simulink model "roll_ap_rev"  (R2021b)
settings: Solver=FixedStepDiscrete  StartTime=0.0  StopTime=25  FixedStep=1/40  RelTol=1e-3
model workspace (MAT data in the model file):
  AP_Eng = [1 1 1 1 1 1 1 1 1 1 1 1 ... (1001 elements, 1001x1)]
  Ail_cmd = [0 -0.149968761714 -0.301000114013 -0.452906745732 -0.6055025668 -0.758604051758 -0.912031519861 -1.0656103303 -1.21917197401 -1.37255504699 -1.52560609378 -1.67818031361 ... (1001 elements, 1001x1)]
  FR = [0; 0; 0; 0; 0; 0]
  HDG_Mode = [0 0 0 0 0 0 0 0 0 0 0 0 ... (1001 elements, 1001x1)]
  HDG_Ref = [0 0 0 0 0 0 0 0 0 0 0 0 ... (1001 elements, 1001x1)]
  InputSize = 6
  N = 28
  P = [0 0 0 0 0 0 0 0 0 0 0 0 ... (1001 elements, 1001x1)]
  Phi = [0 0.0499895872378 0.0999167914439 0.149719695422 0.199337304982 0.248709989094 0.297779895219 0.346491332905 0.3947911197 0.442628884696 0.489957326254 0.536732421812 ... (1001 elements, 1001x1)]
  Psi = [0 0 0 0 0 0 0 0 0 0 0 0 ... (1001 elements, 1001x1)]
  TAS = [0 0 0 0 0 0 0 0 0 0 0 0 ... (1001 elements, 1001x1)]
  TimeSteps = 1001
  TurnK = [0 0 0 0 0 0 0 0 0 0 0 0 ... (1001 elements, 1001x1)]
  X = [-123.259290596  -128.902651481  56.0666516964  743.094931803  83.0616505427  1  -22.0520305237  -100.36159472; 167.816750695  -28.1659382545  59.9981123607  743.132468125  0  1  -48.3367940279  -4.89724193602; 164.580101367  -126.393552121  54.8898007227  346.111605096  0  11.0421280531  95.5860437336  13.049515342; -5.26476645978  105.176372028  156.237569193  657.090475075  0  1  106.271964409  18.5100430761; 109.697619539  165.417273501  -162.797252325  171.186687812  0  1  -112.72586236  193.817894952; -123.259290596  147.137423095  126.863401086  757.740130578  0  1  -22.0520305237  -15.0695729805]
  curPath = '/Users/khouloud.gaaloul/Documents/Projects/QRA-Search/Problems/SimulinkTesting'
  dispGain = Simulink.Parameter
  dispGain.Value = 1
  dispGain.DataType = 'auto'
  dispGain.Complexity = 'real'
  dispGain.Dimensions = [1 1]
  hdgGain = Simulink.Parameter
  hdgGain.Value = 0.015
  hdgGain.DataType = 'auto'
  hdgGain.Min = 0
  hdgGain.Complexity = 'real'
  hdgGain.Dimensions = [1 1]
  hws : handle (value not decoded)
  i = 17
  intGain = Simulink.Parameter
  intGain.Value = 1
  intGain.DataType = 'auto'
  intGain.Complexity = 'real'
  intGain.Dimensions = [1 1]
  j = 4
  list(1).name = 'AP_Eng'
  list(1).size = [1001 1]
  list(1).bytes = 1001
  list(1).class = 'logical'
  list(1).global = 0
  list(1).sparse = 0
  list(1).complex = 0
  list(1).nesting.function = 'simroll_ap'
  list(1).nesting.level = 1
  list(1).persistent = 0
  list(2).name = 'Ail_cmd'
  list(2).size = [1001 1]
  list(2).bytes = 8008
  list(2).class = 'double'
  list(2).global = 0
  list(2).sparse = 0
  list(2).complex = 0
  list(2).nesting.function = 'simroll_ap'
  list(2).nesting.level = 1
  list(2).persistent = 0
  list(3).name = 'FR'
  list(3).size = [6 1]
  list(3).bytes = 48
  list(3).class = 'double'
  list(3).global = 0
  list(3).sparse = 0
  list(3).complex = 0
  list(3).nesting.function = 'simroll_ap'
  list(3).nesting.level = 1
  list(3).persistent = 0
  list(4).name = 'HDG_Mode'
  list(4).size = [1001 1]
  list(4).bytes = 1001
  list(4).class = 'logical'
  list(4).global = 0
  list(4).sparse = 0
  list(4).complex = 0
  list(4).nesting.function = 'simroll_ap'
  list(4).nesting.level = 1
  list(4).persistent = 0
  list(5).name = 'HDG_Ref'
  list(5).size = [1001 1]
  list(5).bytes = 8008
  list(5).class = 'double'
  list(5).global = 0
  list(5).sparse = 0
  list(5).complex = 0
  list(5).nesting.function = 'simroll_ap'
  list(5).nesting.level = 1
  list(5).persistent = 0
  list(6).name = 'InputSize'
  list(6).size = [1 1]
  list(6).bytes = 8
  list(6).class = 'double'
  list(6).global = 0
  list(6).sparse = 0
  list(6).complex = 0
  list(6).nesting.function = 'simroll_ap'
  list(6).nesting.level = 1
  list(6).persistent = 0
  list(7).name = 'N'
  list(7).size = [1 1]
  list(7).bytes = 8
  list(7).class = 'double'
  list(7).global = 0
  list(7).sparse = 0
  list(7).complex = 0
  list(7).nesting.function = 'simroll_ap'
  list(7).nesting.level = 1
  list(7).persistent = 0
  list(8).name = 'P'
  list(8).size = [1001 1]
  list(8).bytes = 8008
  list(8).class = 'double'
  list(8).global = 0
  list(8).sparse = 0
  list(8).complex = 0
  list(8).nesting.function = 'simroll_ap'
  list(8).nesting.level = 1
  list(8).persistent = 0
  list(9).name = 'Phi'
  list(9).size = [1001 1]
  list(9).bytes = 8008
  list(9).class = 'double'
  list(9).global = 0
  list(9).sparse = 0
  list(9).complex = 0
  list(9).nesting.function = 'simroll_ap'
  list(9).nesting.level = 1
  list(9).persistent = 0
  list(10).name = 'Psi'
  list(10).size = [1001 1]
  list(10).bytes = 8008
  list(10).class = 'double'
  list(10).global = 0
  list(10).sparse = 0
  list(10).complex = 0
  list(10).nesting.function = 'simroll_ap'
  list(10).nesting.level = 1
  list(10).persistent = 0
  list(11).name = 'TAS'
  list(11).size = [1001 1]
  list(11).bytes = 8008
  list(11).class = 'double'
  list(11).global = 0
  list(11).sparse = 0
  list(11).complex = 0
  list(11).nesting.function = 'simroll_ap'
  list(11).nesting.level = 1
  list(11).persistent = 0
  list(12).name = 'TimeSteps'
  list(12).size = [1 1]
  list(12).bytes = 8
  list(12).class = 'double'
  list(12).global = 0
  list(12).sparse = 0
  list(12).complex = 0
  list(12).nesting.function = 'simroll_ap'
  list(12).nesting.level = 1
  list(12).persistent = 0
  list(13).name = 'TurnK'
  list(13).size = [1001 1]
  list(13).bytes = 8008
  list(13).class = 'double'
  list(13).global = 0
  list(13).sparse = 0
  list(13).complex = 0
  list(13).nesting.function = 'simroll_ap'
  list(13).nesting.level = 1
  list(13).persistent = 0
  list(14).name = 'X'
  list(14).size = [6 8]
  list(14).bytes = 384
  list(14).class = 'double'
  list(14).global = 0
  list(14).sparse = 0
  list(14).complex = 0
  list(14).nesting.function = 'simroll_ap'
  list(14).nesting.level = 1
  list(14).persistent = 0
  list(15).name = 'curPath'
  list(15).size = [1 78]
  list(15).bytes = 156
  list(15).class = 'char'
  list(15).global = 0
  list(15).sparse = 0
  list(15).complex = 0
  list(15).nesting.function = 'simroll_ap'
  list(15).nesting.level = 1
  list(15).persistent = 0
  list(16).name = 'hws'
  list(16).size = [1 1]
  list(16).bytes = 0
  list(16).class = 'Simulink.ModelWorkspace'
  list(16).global = 0
  list(16).sparse = 0
  list(16).complex = 0
  list(16).nesting.function = 'simroll_ap'
  list(16).nesting.level = 1
  list(16).persistent = 0
  list(17).name = 'i'
  list(17).size = [1 1]
  list(17).bytes = 8
  list(17).class = 'double'
  list(17).global = 0
  list(17).sparse = 0
  list(17).complex = 0
  list(17).nesting.function = 'simroll_ap'
  list(17).nesting.level = 1
  list(17).persistent = 0
  list(18).name = 'j'
  list(18).size = [1 1]
  list(18).bytes = 8
  list(18).class = 'double'
  list(18).global = 0
  list(18).sparse = 0
  list(18).complex = 0
  list(18).nesting.function = 'simroll_ap'
  list(18).nesting.level = 1
  list(18).persistent = 0
  list(19).name = 'list'
  list(19).size = [28 1]
  list(19).bytes = 40880
  list(19).class = 'struct'
  list(19).global = 0
  list(19).sparse = 0
  list(19).complex = 0
  list(19).nesting.function = 'simroll_ap'
  list(19).nesting.level = 1
  list(19).persistent = 0
  list(20).name = 'modelpath'
  list(20).size = [1 95]
  list(20).bytes = 190
  list(20).class = 'char'
  list(20).global = 0
  list(20).sparse = 0
  list(20).complex = 0
  list(20).nesting.function = 'simroll_ap'
  list(20).nesting.level = 1
  list(20).persistent = 0
  list(21).name = 'models'
  list(21).size = [1 4]
  list(21).bytes = 1328
  list(21).class = 'cell'
  list(21).global = 0
  list(21).sparse = 0
  list(21).complex = 0
  list(21).nesting.function = 'simroll_ap'
  list(21).nesting.level = 1
  list(21).persistent = 0
  list(22).name = 'n'
  list(22).size = [1 1]
  list(22).bytes = 8
  list(22).class = 'double'
  list(22).global = 0
  list(22).sparse = 0
  list(22).complex = 0
  list(22).nesting.function = 'simroll_ap'
  list(22).nesting.level = 1
  list(22).persistent = 0
  list(23).name = 'nbrInputs'
  list(23).size = [1 1]
  list(23).bytes = 8
  list(23).class = 'double'
  list(23).global = 0
  list(23).sparse = 0
  list(23).complex = 0
  list(23).nesting.function = 'simroll_ap'
  list(23).nesting.level = 1
  list(23).persistent = 0
  list(24).name = 'rollIn'
  list(24).size = [1 1]
  list(24).bytes = 60394
  list(24).class = 'struct'
  list(24).global = 0
  list(24).sparse = 0
  list(24).complex = 0
  list(24).nesting.function = 'simroll_ap'
  list(24).nesting.level = 1
  list(24).persistent = 0
  list(25).name = 'rollOut'
  list(25).size = [1 1]
  list(25).bytes = 17110
  list(25).class = 'struct'
  list(25).global = 0
  list(25).sparse = 0
  list(25).complex = 0
  list(25).nesting.function = 'simroll_ap'
  list(25).nesting.level = 1
  list(25).persistent = 0
  list(26).name = 's1'
  list(26).size = [1 1001]
  list(26).bytes = 8008
  list(26).class = 'double'
  list(26).global = 0
  list(26).sparse = 0
  list(26).complex = 0
  list(26).nesting.function = 'simroll_ap'
  list(26).nesting.level = 1
  list(26).persistent = 0
  list(27).name = 'simOut'
  list(27).size = [1 1]
  list(27).bytes = 23416
  list(27).class = 'Simulink.SimulationOutput'
  list(27).global = 0
  list(27).sparse = 0
  list(27).complex = 0
  list(27).nesting.function = 'simroll_ap'
  list(27).nesting.level = 1
  list(27).persistent = 0
  list(28).name = 't'
  list(28).size = [1 1001]
  list(28).bytes = 8008
  list(28).class = 'double'
  list(28).global = 0
  list(28).sparse = 0
  list(28).complex = 0
  list(28).nesting.function = 'simroll_ap'
  list(28).nesting.level = 1
  list(28).persistent = 0
  modelpath = '/Users/khouloud.gaaloul/Documents/Projects/QRA-Search/SimulinkModels/autopilot_R2013b_workarea/'
  models = {'/Users/khouloud.gaaloul/Documents/Projects/QRA-Search/SimulinkModels/autopilot_R2013b_workarea/AP_Lib.slx', '/Users/khouloud.gaaloul/Documents/Projects/QRA-Search/SimulinkModels/autopilot_R2013b_workarea/Heading_Mode.slx', '/Users/khouloud.gaaloul/Documents/Projects/QRA-Search/SimulinkModels/autopilot_R2013b_workarea/attitude_controller.slx', '/Users/khouloud.gaaloul/Documents/Projects/QRA-Search/SimulinkModels/autopilot_R2013b_workarea/roll_ap.slx'}
  n = 6
  nbrInputs = 8
  rateGain = Simulink.Parameter
  rateGain.Value = 3
  rateGain.DataType = 'auto'
  rateGain.Complexity = 'real'
  rateGain.Dimensions = [1 1]
  rollIn.signals(1).values = [0 0.0499895872378 0.0999167914439 0.149719695422 0.199337304982 0.248709989094 0.297779895219 0.346491332905 0.3947911197 0.442628884696 0.489957326254 0.536732421812 ... (1001 elements, 1001x1)]
  rollIn.signals(1).dimensions = 1
  rollIn.signals(2).values = [0 0 0 0 0 0 0 0 0 0 0 0 ... (1001 elements, 1001x1)]
  rollIn.signals(2).dimensions = 1
  rollIn.signals(3).values = [0 0 0 0 0 0 0 0 0 0 0 0 ... (1001 elements, 1001x1)]
  rollIn.signals(3).dimensions = 1
  rollIn.signals(4).values = [0 0 0 0 0 0 0 0 0 0 0 0 ... (1001 elements, 1001x1)]
  rollIn.signals(4).dimensions = 1
  rollIn.signals(5).values = [1 1 1 1 1 1 1 1 1 1 1 1 ... (1001 elements, 1001x1)]
  rollIn.signals(5).dimensions = 1
  rollIn.signals(6).values = [0 0 0 0 0 0 0 0 0 0 0 0 ... (1001 elements, 1001x1)]
  rollIn.signals(6).dimensions = 1
  rollIn.signals(7).values = [0 0 0 0 0 0 0 0 0 0 0 0 ... (1001 elements, 1001x1)]
  rollIn.signals(7).dimensions = 1
  rollIn.signals(8).values = [0 0 0 0 0 0 0 0 0 0 0 0 ... (1001 elements, 1001x1)]
  rollIn.signals(8).dimensions = 1
  rollIn.time = [0 0.025 0.05 0.075 0.1 0.125 0.15 0.175 0.2 0.225 0.25 0.275 ... (1001 elements, 1001x1)]
  rollOut.time = [0 0.025 0.05 0.075 0.1 0.125 0.15 0.175 0.2 0.225 0.25 0.275 ... (1001 elements, 1001x1)]
  rollOut.signals.values = [0 -0.149968761714 -0.301000114013 -0.452906745732 -0.6055025668 -0.758604051758 -0.912031519861 -1.0656103303 -1.21917197401 -1.37255504699 -1.52560609378 -1.67818031361 ... (1001 elements, 1001x1)]
  rollOut.signals.dimensions = 1
  rollOut.signals.label = ''
  rollOut.signals.blockName = 'roll_ap/Ail Cmd'
  s1 = [-123.259290596 -123.259290596 -123.259290596 -123.259290596 -123.259290596 -123.259290596 -123.259290596 -123.259290596 -123.259290596 -123.259290596 -123.259290596 -123.259290596 ... (1001 elements, 1x1001)]
  s5 = [0 0 0 0 0 0 0 0 0 0 0 0 ... (1001 elements, 1x1001)]
  simOut = Simulink.SimulationOutput
  simOut.Data.rollOut.time = [0 0.025 0.05 0.075 0.1 0.125 0.15 0.175 0.2 0.225 0.25 0.275 ... (1001 elements, 1001x1)]
  simOut.Data.rollOut.signals.values = [0 -0.149968761714 -0.301000114013 -0.452906745732 -0.6055025668 -0.758604051758 -0.912031519861 -1.0656103303 -1.21917197401 -1.37255504699 -1.52560609378 -1.67818031361 ... (1001 elements, 1001x1)]
  simOut.Data.rollOut.signals.dimensions = 1
  simOut.Data.rollOut.signals.label = ''
  simOut.Data.rollOut.signals.blockName = 'roll_ap/Ail Cmd'
  simOut.Metadata = Simulink.SimulationMetadata
  simOut.Metadata.ModelInfo.ModelName = 'roll_ap'
  simOut.Metadata.ModelInfo.ModelVersion = '1.169'
  simOut.Metadata.ModelInfo.ModelFilePath = '/Users/khouloud.gaaloul/Documents/Projects/QRA-Search/SimulinkModels/autopilot_R2013b_workarea/roll_ap.slx'
  simOut.Metadata.ModelInfo.UserID = 'khouloud.gaaloul'
  simOut.Metadata.ModelInfo.MachineName = ''
  simOut.Metadata.ModelInfo.Platform = 'MACI64'
  simOut.Metadata.ModelInfo.ModelStructuralChecksum = [2583199931; 2424133270; 1270005224; 292482032]
  simOut.Metadata.ModelInfo.SimulationMode = 'normal'
  simOut.Metadata.ModelInfo.StartTime = 0
  simOut.Metadata.ModelInfo.StopTime = 25
  simOut.Metadata.ModelInfo.SolverInfo.Type = 'Fixed-Step'
  simOut.Metadata.ModelInfo.SolverInfo.Solver = 'FixedStepDiscrete'
  simOut.Metadata.ModelInfo.SolverInfo.FixedStepSize = 0.025
  simOut.Metadata.ModelInfo.SimulinkVersion.Name = 'Simulink'
  simOut.Metadata.ModelInfo.SimulinkVersion.Version = '8.7'
  simOut.Metadata.ModelInfo.SimulinkVersion.Release = '(R2016a)'
  simOut.Metadata.ModelInfo.SimulinkVersion.Date = '10-Feb-2016'
  simOut.Metadata.TimingInfo.WallClockTimestampStart = '2018-03-29 14:31:33.008650'
  simOut.Metadata.TimingInfo.WallClockTimestampStop = '2018-03-29 14:31:35.732856'
  simOut.Metadata.TimingInfo.InitializationElapsedWallTime = 2.646185
  simOut.Metadata.TimingInfo.ExecutionElapsedWallTime = 0.010666
  simOut.Metadata.TimingInfo.TerminationElapsedWallTime = 0.067366
  simOut.Metadata.TimingInfo.TotalElapsedWallTime = 2.724217
  simOut.Metadata.ExecutionInfo.StopEvent = 'ReachedStopTime'
  simOut.Metadata.ExecutionInfo.StopEventSource = []
  simOut.Metadata.ExecutionInfo.StopEventDescription = 'Reached stop time of 25'
  simOut.Metadata.ExecutionInfo.ErrorDiagnostic = []
  simOut.Metadata.ExecutionInfo.WarningDiagnostics = struct([])
  simOut.Metadata.AppInfo = struct()
  t = [0 0.025 0.05 0.075 0.1 0.125 0.15 0.175 0.2 0.225 0.25 0.275 ... (1001 elements, 1x1001)]
libraries: simulink x2
(part 1 of 2)
settings Model: RequirementInfo={} %GIDa_fe9045fd_0412_4b6e_8206_617cc20e6fde  ParameterArgumentNames=dispGain,intGain,rateGain,hdgGain  Creator=bpotter  LastModifiedBy=achan260
settings SolverCC: AlgebraicLoopSolver=TrustRegion
settings DataIOCC: ExternalInput=rollIn  LoadExternalInput=on  SaveFormat=StructureWithTime  SaveOutput=off  DSMLogging=off  SaveTime=off  ReturnWorkspaceOutputs=off  OutputSaveName=Ail_Cmd  SignalLoggingName=roll_ap_logsout
settings OptimizationCC: BlockReduction=off  DefaultParameterBehavior=Inlined  InlineInvariantSignals=on  ExpressionDepthLimit=2147483647  EfficientFloat2IntCast=on  EfficientMapNaN2IntZero=off  LifeSpan=inf  MaxStackSize=inf  EfficientTunableParamExpr=on
settings DebuggingCC: SignalInfNanChecking=error  SignalRangeChecking=error  ReadBeforeWriteMsg=EnableAllAsError  WriteAfterWriteMsg=EnableAllAsError  WriteAfterReadMsg=EnableAllAsError  AlgebraicLoopMsg=error  ArtificialAlgebraicLoopMsg=error  SaveWithDisabledLinksMsg=error  SaveWithParameterizedLinksMsg=error  CheckExecutionContextPreStartOutputMsg=on  BlockPriorityViolationMsg=error  MaxConsecutiveZCsMsg=warning  SolverPrmCheckMsg=error  InheritedTsInSrcMsg=error  SingleTaskRateTransMsg=error  TasksWithSamePriorityMsg=error  SigSpecEnsureSampleTimeMsg=error  CheckMatrixSingularityMsg=error  IntegerOverflowMsg=error  ParameterUnderflowMsg=error  ParameterPrecisionLossMsg=error  ParameterTunabilityLossMsg=error  UnderSpecifiedDataTypeMsg=error  UnnecessaryDatatypeConvMsg=warning  VectorMatrixConversionMsg=error  SignalLabelMismatchMsg=error  UnconnectedInputMsg=error  UnconnectedOutputMsg=error  UnconnectedLineMsg=error  SFcnCompatibilityMsg=error  UniqueDataStoreMsg=error  BusObjectLabelMismatch=error  RootOutportRequireBusObject=error  AssertControl=DisableAll  ModelReferenceIOMsg=error  ModelReferenceIOMismatchMessage=error  UnknownTsInhSupMsg=error  ModelReferenceDataLoggingMessage=error  ModelReferenceExtraNoncontSigs=none  StateNameClashWarn=warning  StrictBusMsg=ErrorOnBusTreatedAsVector  NonBusSignalsTreatedAsBus=error  SFUnexpectedBacktrackingDiag=warning  SFNoUnconditionalDefaultTransitionDiag=warning  SFMachineParentedDataDiag=warning  IntegerSaturationMsg=error  ArithmeticOperatorsInVariantConditions=warning
settings HardwareCC: ProdBitPerPointer=32  ProdBitPerSizeT=32  ProdBitPerPtrDiffT=32  ProdLargestAtomicFloat=None  ProdEndianess=BigEndian  ProdWordSize=32  ProdHWDeviceType=32-bit Embedded Processor  TargetHWDeviceType=32-bit Generic
settings ModelReferenceCC: PropagateSignalLabelsOutOfModel=off
settings SFSimCC: SimUseLocalCustomCode=off  MATLABDynamicMemAlloc=off  CustomCodeUndefinedFunction=UseInterfaceOnly
settings RTWCC: Description=Embedded Coder  SystemTargetFile=ert.tlc  TemplateMakefile=ert_default_tmf  GenerateReport=on  RTWVerbose=off  RTWUseLocalCustomCode=off  IncludeHyperlinkInReport=on  LaunchReport=on  PortableWordSizes=on  GenerateTraceInfo=on  GenerateTraceReport=on  GenerateTraceReportSl=on  GenerateTraceReportSf=on  GenerateTraceReportEml=on
settings CodeAppCC: ForceParamTrailComments=on  IgnoreCustomStorageClasses=off  MaxIdLength=63  MangleLength=4  CustomSymbolStrType=$N$R$M  StateflowObjectComments=on  InternalIdentifier=Classic  ReqsInCode=on
settings ERTTargetCC: UtilityFuncGeneration=Shared location  MultiwordLength=2048  IncludeMdlTerminateFcn=off  SuppressErrorStatus=on  SupportAbsoluteTime=off  SupportNonFinite=off  SupportComplex=off  ParenthesesLevel=Maximum  MultiInstanceErrorCode=None  ERTCustomFileTemplate=example_file_process.tlc  PreserveExpressionOrder=on  PreserveIfCondition=on  ConvertIfToSwitch=off  SuppressUnreachableDefaultCases=off
settings ConfigComp: CovSaveName=covdata_rollAP  CovMetricSettings=dcmtrzoiwe  CovHTMLOptions=-sRT=1 -aTS=1 -bRG=1 -bTC=1 -hTR=1 -nFC=0 -scm=1 -bcm=1 -xEv=0  CovSaveCumulativeToWorkspaceVar=on  CovCumulativeVarName=covCumulativeData_rollAP  CovCumulativeReport=on  CovReportOnPause=off  CovExternalEMLEnable=off  PSOpenProjectManager=on  PSSendToPolyspaceServer=on  PSModelRefVerifDepth=All  PSAutoStubLUT=off  DVMakeOutputFilesUnique=off  DVMaxTestCaseSteps=500  DVTestSuiteOptimization=CombinedObjectives (Nonlinear Extended)  DVDetectActiveLogic=on  DVSaveHarnessModel=on  DVModelReferenceHarness=on  DVSaveReport=on

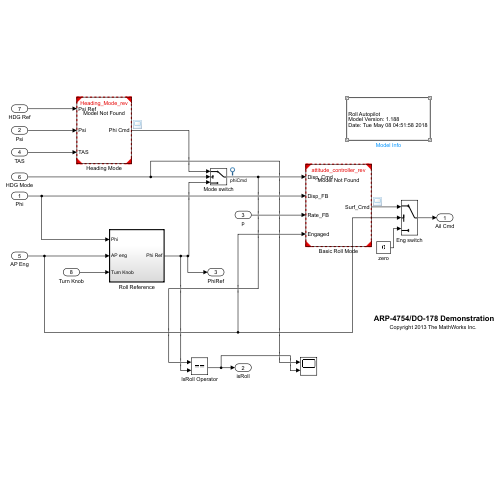
[thumbnail: Simulink's stored preview of the top-level diagram]
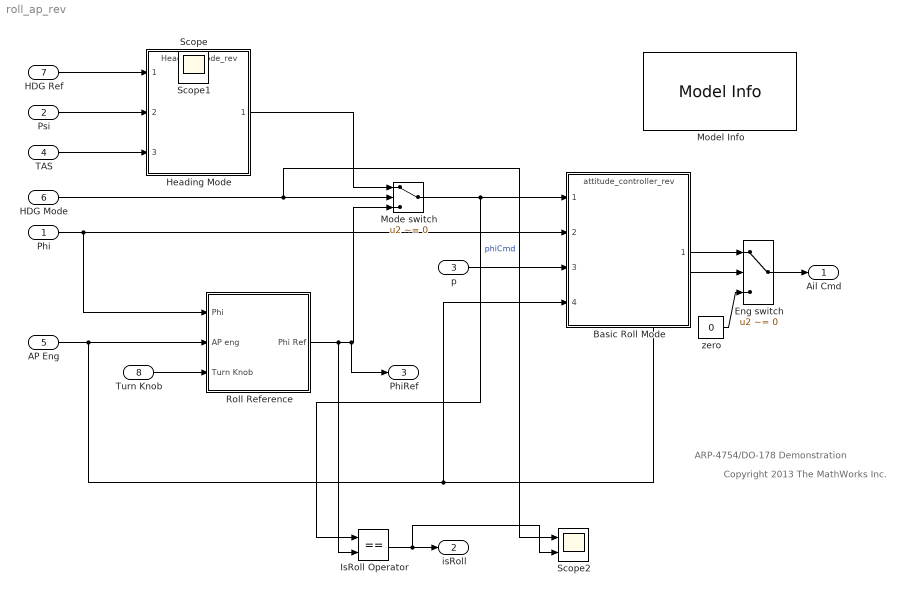
== system roll_ap_rev ==
  note: Copyright 2013 The MathWorks Inc.
  note: ARP-4754/DO-178 Demonstration
  Phi : Inport  RequirementInfo={'other' 'do178b_autopilot_requirements.docx' '@Simulink_requirement_item_3' 'true' '1.3. Roll Hold Reference' ' ' ; 'other' 'do178b_autopilot_requirements.docx' '@Simulink_requirement_item_4' 'true' '1.4. Roll Performance' '' } %GIDa_040c2d73_6311_42f9_964f_56f1fff3d8d8  OutMin=-180  OutMax=180  OutDataTypeStr=double  PortDimensions=1  SampleTime=1/40  Interpolate=off
  Psi : Inport  RequirementInfo={'other' 'do178b_autopilot_requirements.docx' '@Simulink_requirement_item_10' 'true' '1.10. Heading Performance' '' } %GIDa_aa699f91_96f0_401b_acdb_f9b4b0743533  Port=2  OutMin=-180  OutMax=180  OutDataTypeStr=double  PortDimensions=1  SampleTime=1/40  Interpolate=off
  p : Inport  RequirementInfo={'other' 'do178b_autopilot_requirements.docx' '@Simulink_requirement_item_4' 'true' '1.4. Roll Performance' '' } %GIDa_91b6e343_cedd_4c09_9e82_9cc09e4312a7  Port=3  OutMin=-180  OutMax=180  OutDataTypeStr=double  PortDimensions=1  SampleTime=1/40  Interpolate=off
  TAS : Inport  RequirementInfo={'other' 'do178b_autopilot_requirements.docx' '@Simulink_requirement_item_10' 'true' '1.10. Heading Performance' '' } %GIDa_9daa2c3d_09c1_4ac6_a206_1425f5f778cd  Port=4  OutMin=0  OutMax=1000  OutDataTypeStr=double  PortDimensions=1  SampleTime=1/40  Interpolate=off
  AP Eng : Inport  RequirementInfo={'other' 'do178b_autopilot_requirements.docx' '@Simulink_requirement_item_1' 'true' '1.1. Roll Autopilot Engage Control' ' ' ; 'other' 'do178b_autopilot_requirements.docx' '@Simulink_requirement_item_3' 'true' '1.3. Roll Hold Reference' ' ' ; 'other' 'do178b_autopilot_requirements.docx' '@Simulink_requirement_item_4' 'true' '1.4. Roll Performance' '' } %GIDa_dbf8c750_871c_42fc_8ea1_57838e97fa97  Port=5  OutDataTypeStr=boolean  PortDimensions=1  SampleTime=1/40  Interpolate=off
  HDG Mode : Inport  RequirementInfo={'other' 'do178b_autopilot_requirements.docx' '@Simulink_requirement_item_2' 'true' '1.2. Roll Hold Mode' ' ' ; 'other' 'do178b_autopilot_requirements.docx' '@Simulink_requirement_item_8' 'true' '1.8. Heading Hold Mode' '' } %GIDa_3d1fd2be_b046_42ef_8f3c_1955bceadbb7  Port=6  OutDataTypeStr=boolean  PortDimensions=1  SampleTime=1/40  Interpolate=off
  HDG Ref : Inport  RequirementInfo={'other' 'do178b_autopilot_requirements.docx' '@Simulink_requirement_item_9' 'true' '1.9. Heading Hold Reference' ' ' ; 'other' 'do178b_autopilot_requirements.docx' '@Simulink_requirement_item_10' 'true' '1.10. Heading Performance' '' } %GIDa_96162cda_cb1a_490e_8dac_f861526aad50  Port=7  OutMin=-180  OutMax=180  OutDataTypeStr=double  PortDimensions=1  SampleTime=1/40  Interpolate=off
  Turn Knob : Inport  RequirementInfo={'other' 'do178b_autopilot_requirements.docx' '@Simulink_requirement_item_3' 'true' '1.3. Roll Hold Reference' '' } %GIDa_fa976ccd_1ea9_4823_b673_fef2768ad601  Port=8  OutMin=-45  OutMax=45  OutDataTypeStr=double  PortDimensions=1  SampleTime=1/40  Interpolate=off
  Basic Roll Mode : ModelReference  RequirementInfo={'other' 'do178b_autopilot_requirements.docx' '@Simulink_requirement_item_4' 'true' '1.4. Roll Performance' '' ; 'other' 'do178b_autopilot_requirements.docx' '@Simulink_requirement_item_5' 'true' '1.5. Roll Rate Limit' '' ; 'other' 'do178b_autopilot_requirements.docx' '@Simulink_requirement_item_6' 'true' '1.6. Roll Angle Limit' '' ; 'other' 'do178b_autopilot_requirements.docx' '@Simulink_requirement_item_7' 'true' '1.7. Aileron Angle Limit' '' } %GIDa_94fed7b0_f432_43f5_a2d9_2abccf075f5b  ModelNameDialog=attitude_controller_rev  SimulationMode=Normal  ModelReferenceVersion=1.70
  Eng switch : Switch  RequirementInfo={'other' 'do178b_autopilot_requirements.docx' '' 'true' '1.1. Roll Autopilot Engage Control' ' ' } %GIDa_1f89e2a1_f10b_411b_80f1_4c7070559f04  Criteria=u2 ~= 0
  Heading Mode : ModelReference  RequirementInfo={'other' 'do178b_autopilot_requirements.docx' '@Simulink_requirement_item_10' 'true' '1.10. Heading Performance' '' } %GIDa_e0954c89_e814_46d2_8f67_6d4b1cdfab81  ModelNameDialog=Heading_Mode_rev  SimulationMode=Normal  ModelReferenceVersion=1.148
  "IsRoll Operator " : RelationalOperator  Operator===  OutDataTypeStr=boolean  RndMeth=Nearest
  Mode switch : Switch  RequirementInfo={'other' 'do178b_autopilot_requirements.docx' '@Simulink_requirement_item_2' 'true' '1.2. Roll Hold Mode' ' ' ; 'other' 'do178b_autopilot_requirements.docx' '@Simulink_requirement_item_4' 'true' '1.4. Roll Performance' ' ' ; 'other' 'do178b_autopilot_requirements.docx' '@Simulink_requirement_item_8' 'true' '1.8. Heading Hold Mode' ' ' ; 'other' 'do178b_autopilot_requirements.docx' '@Simulink_requirement_item_10' 'true' '1.10. Heading Performance' '' } %GIDa_89518de0_411a_4ee8_869d_c7ed5e5087e3  Criteria=u2 ~= 0
  Model Info : simulink/Model-Wide Utilities/Model Info  RequirementInfo={} %GIDa_ca11a4b2_f22f_461f_8532_eb2c7aa53101  Frame=on  DisplayStringWithTags=|  HorizontalTextAlignment=Left  LeftAlignmentValue=0.02
      | Roll Autopilot
      | Model Version: %<ModelVersion>
      | Date: %<LastModificationDate>
  Roll Reference : Subsystem  RequirementInfo={'other' 'do178b_autopilot_requirements.docx' '@Simulink_requirement_item_3' 'true' '1.3. Roll Hold Reference' '' } %GIDa_c8cf196e_df7c_4434_8b0c_5575b514a7cf  TreatAsAtomicUnit=on
      settings: RTWSystemCode=Inline
  Scope2 : Scope  NumInputPorts=2
  zero : Constant  RequirementInfo={'other' 'do178b_autopilot_requirements.docx' '' 'true' '1.1. Roll Autopilot Engage Control' '' } %GIDa_8c99e557_6257_4659_beae_770a67a6ac3a  Value=0  OutDataTypeStr=double
  Ail Cmd : Outport  RequirementInfo={'other' 'do178b_autopilot_requirements.docx' '' 'true' '1.1. Roll Autopilot Engage Control' ' ' } %GIDa_02b61f6d_71d4_4b0d_89ac_bfbca808eb5f  OutDataTypeStr=double  PortDimensions=1  SampleTime=1/40
  isRoll : Outport  Port=2
  PhiRef : Outport  Port=3
  Scope : Scope
  Scope1 : Scope
  wires:
  HDG Ref/1 -> Heading Mode/1
  Phi/1 -> Roll Reference/1(Phi), Basic Roll Mode/2
  p/1 -> Basic Roll Mode/3
  Psi/1 -> Heading Mode/2
  TAS/1 -> Heading Mode/3
  Mode switch/1 -> "IsRoll Operator "/1, Basic Roll Mode/1  "phiCmd"
  HDG Mode/1 -> Scope2/1, Mode switch/2
  AP Eng/1 -> Eng switch/2, Basic Roll Mode/4, Roll Reference/2(AP eng)
  Basic Roll Mode/1 -> Eng switch/1
  Eng switch/1 -> Ail Cmd/1
  zero/1 -> Eng switch/3
  Roll Reference/1(Phi Ref) -> "IsRoll Operator "/2, PhiRef/1, Mode switch/3
  Turn Knob/1 -> Roll Reference/3(Turn Knob)
  Heading Mode/1 -> Mode switch/1
  "IsRoll Operator "/1 -> Scope2/2, isRoll/1
